simulink model "MotorSim"  (R2024b)
settings: Solver=VariableStepAuto  StartTime=0.0  StopTime=100  RelTol=1e-3
libraries: dc_motor_lib x1

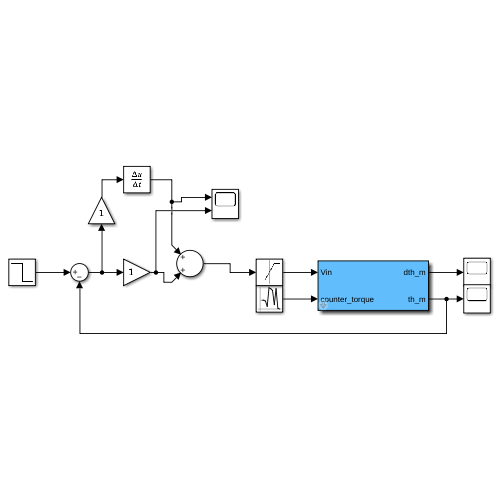
[thumbnail: Simulink's stored preview of the top-level diagram]
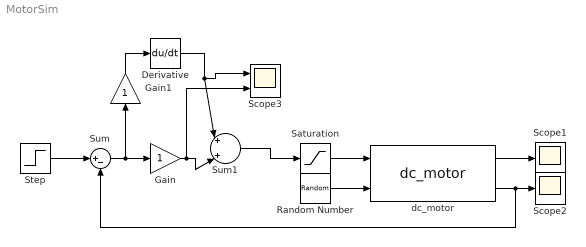
== system MotorSim ==
  Derivative : Derivative
  Gain : Gain
  Gain1 : Gain
  Random Number : RandomNumber  Variance=0.005  SampleTime=0.1
  Saturation : Saturate  UpperLimit=1  LowerLimit=-1
  Scope1 : Scope
  Scope2 : Scope
  Scope3 : Scope  NumInputPorts=2
  Step : Step  Time=0  After=-1000  SampleTime=0
  Sum : Sum  Inputs=|+-
  Sum1 : Sum  Inputs=|+|+|
  dc_motor : dc_motor_lib/dc_motor  Rm=1  Lm=0.01  Kb=1/((406*2*pi)/60)  Kt=1  Jm=0.013  bm=0
      settings: SourceProductName=DC Motor Library
  wires:
  dc_motor/1 -> Scope1/1
  Saturation/1 -> dc_motor/1
  Step/1 -> Sum/1
  Sum/1 -> Gain1/1, Gain/1
  dc_motor/2 -> Sum/2, Scope2/1
  Random Number/1 -> dc_motor/2
  Gain1/1 -> Derivative/1
  Gain/1 -> Scope3/2, Sum1/2
  Derivative/1 -> Scope3/1, Sum1/1
  Sum1/1 -> Saturation/1
